simulink model "V2_SIMULINK"  (R2018b)
settings: Solver=VariableStepAuto  StartTime=0.0  StopTime=10.0  RelTol=1e-3
settings Model: Creator=Mieko  LastModifiedBy=Mieko

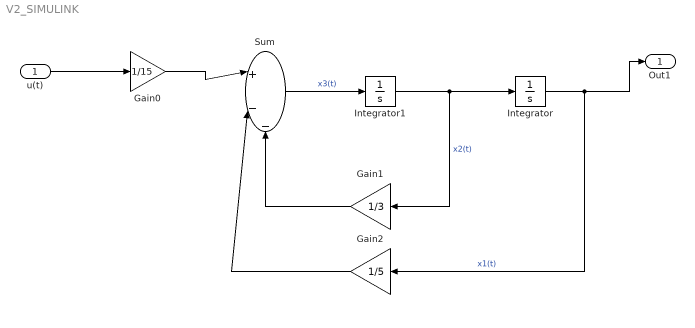
== system V2_SIMULINK ==
  u(t) : Inport
  Gain0 : Gain  Gain=1/15
  Gain1 : Gain  Gain=1/3
  Gain2 : Gain  Gain=1/5
  Integrator : Integrator
  Integrator1 : Integrator
  Sum : Sum  Inputs=|+--
  Out1 : Outport  SignalName=y(t)
  wires:
  Integrator/1 -> Gain2/1, Out1/1  "x1(t)"
  Integrator1/1 -> Gain1/1, Integrator/1  "x2(t)"
  Gain0/1 -> Sum/1
  u(t)/1 -> Gain0/1
  Gain1/1 -> Sum/3
  Sum/1 -> Integrator1/1  "x3(t)"
  Gain2/1 -> Sum/2
